simulink model "Test_Byte_Demultiplexer_1_to_2"  (Simulink 8.1)
settings: Solver=ode45  StartTime=0.0  StopTime=len  RelTol=1e-3
libraries: Byte_Demultiplexers_Lib x1, commutil2 x1
settings Model: Creator=N  LastModifiedBy=uzivatel
settings DataIOCC: LimitDataPoints=off  SignalLoggingSaveFormat=Dataset
settings OptimizationCC: ExpressionDepthLimit=128
settings DebuggingCC: UnderspecifiedInitializationDetection=Simplified  MergeDetectMultiDrivingBlocksExec=error  SolverPrmCheckMsg=none  FcnCallInpInsideContextMsg=EnableAllAsError  FrameProcessingCompatibilityMsg=error  StateNameClashWarn=none
settings HardwareCC: ProdBitPerPointer=64  ProdLargestAtomicFloat=Float  ProdIntDivRoundTo=Zero  ProdEndianess=LittleEndian  ProdHWDeviceType=Intel->x86-64 (Windows64)
settings ModelReferenceCC: PropagateSignalLabelsOutOfModel=on
settings GRTTargetCC: CodeReplacementLibrary=None  CombineOutputUpdateFcns=on  CPPClassGenCompliant=on  GRTInterface=off

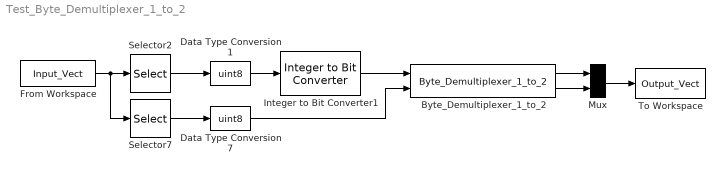
== system Test_Byte_Demultiplexer_1_to_2 ==
  Byte_Demultiplexer_1_to_2 : Byte_Demultiplexers_Lib/Byte_Demultiplexers_Lib/Byte_Demultiplexer_1_to_2
  Data Type Conversion1 : DataTypeConversion  OutDataTypeStr=uint8
  Data Type Conversion7 : DataTypeConversion  OutDataTypeStr=uint8
  From Workspace : FromWorkspace  VariableName=Input_Vect  SampleTime=1  Interpolate=off  OutputAfterFinalValue=Holding final value
  Integer to Bit Converter1 : commutil2/Integer to Bit Converter  nbits=1  signedInputValues=Unsigned  bitOrder=MSB first  outDtype=boolean
  Mux : Mux  Inputs=2
  Selector2 : Selector  IndexMode=Zero-based  InputPortWidth=2  SampleTime=1  IndexOptions=Index vector (dialog)  Indices=0  OutputSizes=1
  Selector7 : Selector  IndexMode=Zero-based  InputPortWidth=2  IndexOptions=Index vector (dialog)  Indices=1  OutputSizes=1
  To Workspace : ToWorkspace  VariableName=Output_Vect  SampleTime=1
  wires:
  Integer to Bit Converter1/1 -> Byte_Demultiplexer_1_to_2/1
  Data Type Conversion1/1 -> Integer to Bit Converter1/1
  Selector2/1 -> Data Type Conversion1/1
  From Workspace/1 -> Selector7/1, Selector2/1
  Data Type Conversion7/1 -> Byte_Demultiplexer_1_to_2/2
  Selector7/1 -> Data Type Conversion7/1
  Byte_Demultiplexer_1_to_2/1 -> Mux/1
  Byte_Demultiplexer_1_to_2/2 -> Mux/2
  Mux/1 -> To Workspace/1
